simulink model "Tavola3_11_FL"  (R2018b)
settings: Solver=FixedStepAuto  StartTime=0.0  StopTime=10.0  RelTol=1e-3
settings Model: Creator=Utente  LastModifiedBy=Utente

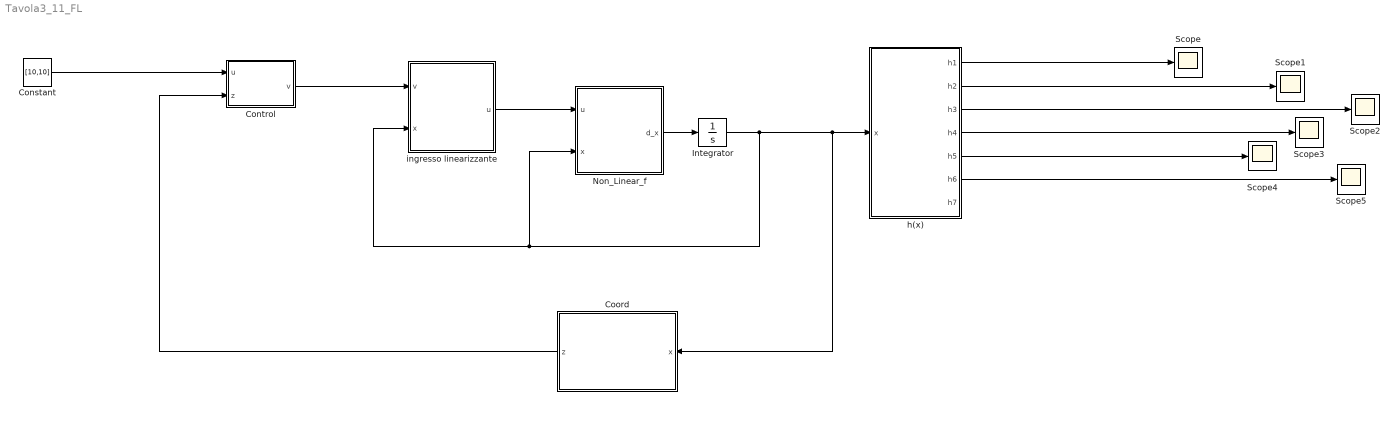
== system Tavola3_11_FL ==
  Constant : Constant  Value=[10,10]
  Control : MATLAB Function  TreatAsAtomicUnit=on
  Coord : MATLAB Function  TreatAsAtomicUnit=on
  Integrator : Integrator  InitialCondition=[0,0,0,0,0,5,0,0]
  "Non_Linear_f " : MATLAB Function  TreatAsAtomicUnit=on
  Scope{,1..5} (6 alike) : Scope
  h(x) : MATLAB Function  TreatAsAtomicUnit=on
  ingresso linearizzante : MATLAB Function  TreatAsAtomicUnit=on
  wires:
  "Non_Linear_f "/1(d_x) -> Integrator/1
  Integrator/1 -> Coord/1(x), h(x)/1(x), ingresso linearizzante/2(x), "Non_Linear_f "/2(x)
  h(x)/1(h1) -> Scope/1
  ingresso linearizzante/1(u) -> "Non_Linear_f "/1(u)
  Control/1(v) -> ingresso linearizzante/1(v)
  h(x)/2(h2) -> Scope1/1
  Constant/1 -> Control/1(u)
  Coord/1(z) -> Control/2(z)
  h(x)/3(h3) -> Scope2/1
  h(x)/4(h4) -> Scope3/1
  h(x)/5(h5) -> Scope4/1
  h(x)/6(h6) -> Scope5/1

== matlab function Tavola3_11_FL/h(x) ==
  data: x input; h1 output; h2 output; h3 output; h4 output; h5 output; h6 output; h7 output
function [h1,h2,h3,h4,h5,h6,h7] = h(x)

x1 = x(1);
x2 = x(2);
x3 = x(3);
x4 = x(4);
x5 = x(5);
x6 = x(6);
x7 = x(7);


h1 = x1;
h2 = x2;
h3 = x3;
h4 = x4;
h5 = x5;
h6 = x6;
h7 = x7;

== matlab function Tavola3_11_FL/Non_Linear_f  ==
  data: u input; d_x output; x input
function d_x = statespacef(u,x)

x1 = x(1);
x2 = x(2);
x3 = x(3);
x4 = x(4);
x5 = x(5);
x6 = x(6);
x7 = x(7);
x8 = x(8);

f =                                                                                                                                                                                                                                                                                                                                                                                          [x6*cos(x3);
                                                                                                                                                                                                                                                                                                                                                                                              x6*sin(x3);
                                                                                                                                                                                                                                                                                                                                                                                                      x7;
                                                                                                                                                                                                                                                                                                                                                                                                      x5;
                                                                                                                                                                                                                                                                                                                                                                                                      x8;
 x7^2*(1.99*sin(3.0*x4) - 6.77*sin(x4)) + (23.5*sin(2.0*x4))/(4.79*cos(x4)^2 - 12.5) - (x8*((35*cos(x4))/64 + 1603/1600))/((35*cos(x3))/16 + 249/80) - (1.0*(0.547*cos(x4) + 1.0)*((3.28*sin(2.0*x4)*x7^2)/(4.79*cos(x4)^2 - 12.5) + (173.0*sin(x4))/(4.79*cos(x4)^2 - 12.5) - (2.39*x5^2*sin(2.0*x4))/(4.79*cos(x4)^2 - 12.5)))/(2.19*cos(x3) + 3.11) - (2.19*x5^2*sin(2.0*x4))/(4.79*cos(x4)^2 - 12.5);
                                                                                                                                                                                                                                                                                                                                                                                                       0;
                                                                                                                                                                                                                                                                                                                                                                                                       0];
                                   
g1_tilde = [zeros(7,1);1];
g2_tilde = [zeros(6,1);1;0];

d_x = f + [g1_tilde,g2_tilde]*u;

== matlab function Tavola3_11_FL/ingresso linearizzante ==
  data: v input; u output; x input
function u = inputLinearizzante(v,x)

x1 = x(1);
x2 = x(2);
x3 = x(3);
x4 = x(4);
x5 = x(5);
x6 = x(6);
x7 = x(7);
x8 = x(8);

Gamma = [x7*sin(x3)*((x8*((35*cos(x4))/64 + 1603/1600))/((35*cos(x3))/16 + 249/80) - (23.5*sin(2.0*x4))/(4.79*cos(x4)^2 - 12.5) - x7^2*(1.99*sin(3.0*x4) - 6.77*sin(x4)) + (1.0*(0.547*cos(x4) + 1.0)*((3.28*sin(2.0*x4)*x7^2)/(4.79*cos(x4)^2 - 12.5) + (173.0*sin(x4))/(4.79*cos(x4)^2 - 12.5) - (2.39*x5^2*sin(2.0*x4))/(4.79*cos(x4)^2 - 12.5)))/(2.19*cos(x3) + 3.11) + (2.19*x5^2*sin(2.0*x4))/(4.79*cos(x4)^2 - 12.5)) - x8*cos(x3)*((4.38*x5*sin(2.0*x4))/(4.79*cos(x4)^2 - 12.5) - (4.79*x5*sin(2.0*x4)*(0.547*cos(x4) + 1.0))/((2.19*cos(x3) + 3.11)*(4.79*cos(x4)^2 - 12.5))) - x7*(cos(x3)*((35*x8*sin(x3)*((35*cos(x4))/64 + 1603/1600))/(16*((35*cos(x3))/16 + 249/80)^2) + (2.19*sin(x3)*(0.547*cos(x4) + 1.0)*((3.28*sin(2.0*x4)*x7^2)/(4.79*cos(x4)^2 - 12.5) + (173.0*sin(x4))/(4.79*cos(x4)^2 - 12.5) - (2.39*x5^2*sin(2.0*x4))/(4.79*cos(x4)^2 - 12.5)))/(2.19*cos(x3) + 3.11)^2) - sin(x3)*((x8*((35*cos(x4))/64 + 1603/1600))/((35*cos(x3))/16 + 249/80) - (23.5*sin(2.0*x4))/(4.79*cos(x4)^2 - 12.5) - x7^2*(1.99*sin(3.0*x4) - 6.77*sin(x4)) + (1.0*(0.547*cos(x4) + 1.0)*((3.28*sin(2.0*x4)*x7^2)/(4.79*cos(x4)^2 - 12.5) + (173.0*sin(x4))/(4.79*cos(x4)^2 - 12.5) - (2.39*x5^2*sin(2.0*x4))/(4.79*cos(x4)^2 - 12.5)))/(2.19*cos(x3) + 3.11) + (2.19*x5^2*sin(2.0*x4))/(4.79*cos(x4)^2 - 12.5)) + x6*x7*cos(x3)) + x5*cos(x3)*(x7^2*(5.98*cos(3.0*x4) - 6.77*cos(x4)) + (46.9*cos(2.0*x4))/(4.79*cos(x4)^2 - 12.5) - (1.0*(0.547*cos(x4) + 1.0)*((173.0*cos(x4))/(4.79*cos(x4)^2 - 12.5) + (1666.0*cos(x4)*sin(x4)^2)/(4.79*cos(x4)^2 - 12.5)^2 - (4.79*x5^2*cos(2.0*x4))/(4.79*cos(x4)^2 - 12.5) + (6.57*x7^2*cos(2.0*x4))/(4.79*cos(x4)^2 - 12.5) - (22.9*x5^2*sin(2.0*x4)*cos(x4)*sin(x4))/(4.79*cos(x4)^2 - 12.5)^2 + (31.4*x7^2*sin(2.0*x4)*cos(x4)*sin(x4))/(4.79*cos(x4)^2 - 12.5)^2))/(2.19*cos(x3) + 3.11) + (0.547*sin(x4)*((3.28*sin(2.0*x4)*x7^2)/(4.79*cos(x4)^2 - 12.5) + (173.0*sin(x4))/(4.79*cos(x4)^2 - 12.5) - (2.39*x5^2*sin(2.0*x4))/(4.79*cos(x4)^2 - 12.5)))/(2.19*cos(x3) + 3.11) - (4.38*x5^2*cos(2.0*x4))/(4.79*cos(x4)^2 - 12.5) + (35*x8*sin(x4))/(64*((35*cos(x3))/16 + 249/80)) + (225.0*sin(2.0*x4)*cos(x4)*sin(x4))/(4.79*cos(x4)^2 - 12.5)^2 - (21.0*x5^2*sin(2.0*x4)*cos(x4)*sin(x4))/(4.79*cos(x4)^2 - 12.5)^2);
         x5*sin(x3)*(x7^2*(5.98*cos(3.0*x4) - 6.77*cos(x4)) + (46.9*cos(2.0*x4))/(4.79*cos(x4)^2 - 12.5) - (1.0*(0.547*cos(x4) + 1.0)*((173.0*cos(x4))/(4.79*cos(x4)^2 - 12.5) + (1666.0*cos(x4)*sin(x4)^2)/(4.79*cos(x4)^2 - 12.5)^2 - (4.79*x5^2*cos(2.0*x4))/(4.79*cos(x4)^2 - 12.5) + (6.57*x7^2*cos(2.0*x4))/(4.79*cos(x4)^2 - 12.5) - (22.9*x5^2*sin(2.0*x4)*cos(x4)*sin(x4))/(4.79*cos(x4)^2 - 12.5)^2 + (31.4*x7^2*sin(2.0*x4)*cos(x4)*sin(x4))/(4.79*cos(x4)^2 - 12.5)^2))/(2.19*cos(x3) + 3.11) + (0.547*sin(x4)*((3.28*sin(2.0*x4)*x7^2)/(4.79*cos(x4)^2 - 12.5) + (173.0*sin(x4))/(4.79*cos(x4)^2 - 12.5) - (2.39*x5^2*sin(2.0*x4))/(4.79*cos(x4)^2 - 12.5)))/(2.19*cos(x3) + 3.11) - (4.38*x5^2*cos(2.0*x4))/(4.79*cos(x4)^2 - 12.5) + (35*x8*sin(x4))/(64*((35*cos(x3))/16 + 249/80)) + (225.0*sin(2.0*x4)*cos(x4)*sin(x4))/(4.79*cos(x4)^2 - 12.5)^2 - (21.0*x5^2*sin(2.0*x4)*cos(x4)*sin(x4))/(4.79*cos(x4)^2 - 12.5)^2) - x8*sin(x3)*((4.38*x5*sin(2.0*x4))/(4.79*cos(x4)^2 - 12.5) - (4.79*x5*sin(2.0*x4)*(0.547*cos(x4) + 1.0))/((2.19*cos(x3) + 3.11)*(4.79*cos(x4)^2 - 12.5))) - x7*cos(x3)*((x8*((35*cos(x4))/64 + 1603/1600))/((35*cos(x3))/16 + 249/80) - (23.5*sin(2.0*x4))/(4.79*cos(x4)^2 - 12.5) - x7^2*(1.99*sin(3.0*x4) - 6.77*sin(x4)) + (1.0*(0.547*cos(x4) + 1.0)*((3.28*sin(2.0*x4)*x7^2)/(4.79*cos(x4)^2 - 12.5) + (173.0*sin(x4))/(4.79*cos(x4)^2 - 12.5) - (2.39*x5^2*sin(2.0*x4))/(4.79*cos(x4)^2 - 12.5)))/(2.19*cos(x3) + 3.11) + (2.19*x5^2*sin(2.0*x4))/(4.79*cos(x4)^2 - 12.5)) - x7*(sin(x3)*((35*x8*sin(x3)*((35*cos(x4))/64 + 1603/1600))/(16*((35*cos(x3))/16 + 249/80)^2) + (2.19*sin(x3)*(0.547*cos(x4) + 1.0)*((3.28*sin(2.0*x4)*x7^2)/(4.79*cos(x4)^2 - 12.5) + (173.0*sin(x4))/(4.79*cos(x4)^2 - 12.5) - (2.39*x5^2*sin(2.0*x4))/(4.79*cos(x4)^2 - 12.5)))/(2.19*cos(x3) + 3.11)^2) + cos(x3)*((x8*((35*cos(x4))/64 + 1603/1600))/((35*cos(x3))/16 + 249/80) - (23.5*sin(2.0*x4))/(4.79*cos(x4)^2 - 12.5) - x7^2*(1.99*sin(3.0*x4) - 6.77*sin(x4)) + (1.0*(0.547*cos(x4) + 1.0)*((3.28*sin(2.0*x4)*x7^2)/(4.79*cos(x4)^2 - 12.5) + (173.0*sin(x4))/(4.79*cos(x4)^2 - 12.5) - (2.39*x5^2*sin(2.0*x4))/(4.79*cos(x4)^2 - 12.5)))/(2.19*cos(x3) + 3.11) + (2.19*x5^2*sin(2.0*x4))/(4.79*cos(x4)^2 - 12.5)) + x6*x7*sin(x3))];
 
E = [ -(cos(x3)*((35*cos(x4))/64 + 1603/1600))/((35*cos(x3))/16 + 249/80), cos(x3)*(2*x7*(1.99*sin(3.0*x4) - 6.77*sin(x4)) - (6.57*x7*sin(2.0*x4)*(0.547*cos(x4) + 1.0))/((2.19*cos(x3) + 3.11)*(4.79*cos(x4)^2 - 12.5))) - x6*sin(x3);
      -(sin(x3)*((35*cos(x4))/64 + 1603/1600))/((35*cos(x3))/16 + 249/80), x6*cos(x3) + sin(x3)*(2*x7*(1.99*sin(3.0*x4) - 6.77*sin(x4)) - (6.57*x7*sin(2.0*x4)*(0.547*cos(x4) + 1.0))/((2.19*cos(x3) + 3.11)*(4.79*cos(x4)^2 - 12.5)))];

inv_E = inv(E);

u = -inv_E*Gamma+inv_E*v;

== matlab function Tavola3_11_FL/Coord ==
  data: x input; z output
function z = transformCoordinate(x)

    x1 = x(1);
    x2 = x(2);
    x3 = x(3);
    x4 = x(4);
    x5 = x(5);
    x6 = x(6);
    x7 = x(7);
    x8 = x(8);

    z = [                                                                                                                                                                                                                                                                                                                                                                                                                            x1;
                                                                                                                                                                                                                                                                                                                                                                                                                              x6*cos(x3);
     - cos(x3)*((x8*((35*cos(x4))/64 + 1603/1600))/((35*cos(x3))/16 + 249/80) - (23.5*sin(2.0*x4))/(4.79*cos(x4)^2 - 12.5) - x7^2*(1.99*sin(3.0*x4) - 6.77*sin(x4)) + (1.0*(0.547*cos(x4) + 1.0)*((3.28*sin(2.0*x4)*x7^2)/(4.79*cos(x4)^2 - 12.5) + (173.0*sin(x4))/(4.79*cos(x4)^2 - 12.5) - (2.39*x5^2*sin(2.0*x4))/(4.79*cos(x4)^2 - 12.5)))/(2.19*cos(x3) + 3.11) + (2.19*x5^2*sin(2.0*x4))/(4.79*cos(x4)^2 - 12.5)) - x6*x7*sin(x3);
                                                                                                                                                                                                                                                                                                                                                                                                                                      x2;
                                                                                                                                                                                                                                                                                                                                                                                                                              x6*cos(x3);
      x6*x7*cos(x3) - sin(x3)*((x8*((35*cos(x4))/64 + 1603/1600))/((35*cos(x3))/16 + 249/80) - (23.5*sin(2.0*x4))/(4.79*cos(x4)^2 - 12.5) - x7^2*(1.99*sin(3.0*x4) - 6.77*sin(x4)) + (1.0*(0.547*cos(x4) + 1.0)*((3.28*sin(2.0*x4)*x7^2)/(4.79*cos(x4)^2 - 12.5) + (173.0*sin(x4))/(4.79*cos(x4)^2 - 12.5) - (2.39*x5^2*sin(2.0*x4))/(4.79*cos(x4)^2 - 12.5)))/(2.19*cos(x3) + 3.11) + (2.19*x5^2*sin(2.0*x4))/(4.79*cos(x4)^2 - 12.5))];
 
 
 

end

== matlab function Tavola3_11_FL/Control ==
  data: u input; z input; v output
function v = control(u,z)
    
    v = zeros(2,1);
    
    k = [-500 30 -500 -500 30 -500];
      
    v(1) = -k(1)*(z(1)-0) -k(2)*(z(2)-0) -k(3)*(z(3)-0);
    v(2) = -k(4)*(z(4)-0) -k(5)*(z(5)-0) -k(6)*(z(3)-0);
    
    
end
